simulink model "SEMS_2025_MATLAB file"  (R2024b)
settings: Solver=VariableStepAuto  StartTime=0.0  StopTime=24  RelTol=1e-3
undefined symbols (not defined in the file): Ion, Lithium
libraries: spsSeriesRLCBranchLib x4, spsBatteryLib x1, spsCurrentMeasurementLib x1, spsDiodeLib x1, spsIGBTDiodeLib x1, spsPVArrayLib x1, spsPWMGeneratorDCDCLib x1, spsVoltageMeasurementLib x1, spspowerguiLib x1
settings Model: Creator=sumanth  LastModifiedBy=sumanth

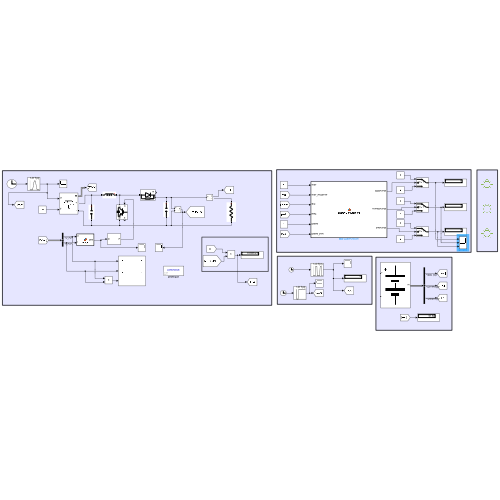
[thumbnail: Simulink's stored preview of the top-level diagram]
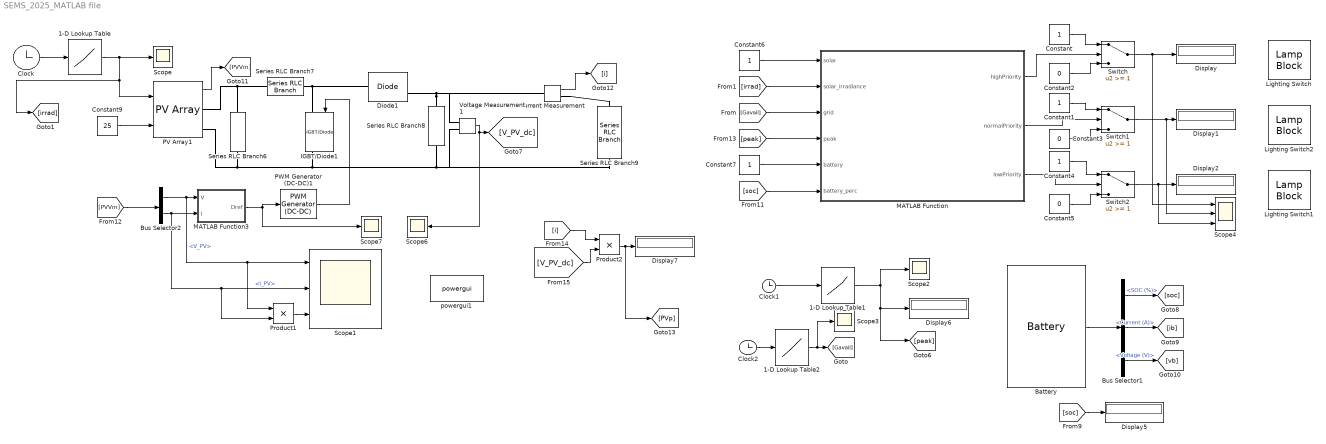
== system SEMS_2025_MATLAB file ==
  1-D Lookup Table : Lookup_n-D  NumberOfTableDimensions=1  BreakpointsForDimension1=[0 1 2 3 4 5 6 7 8 9 10 11 12 13 14 15 16 17 18 19 20 21 22 23]  Table=[0 0 0 0 0 0 0 79 315 533 710 819 855 817 707 532 311 75 0 0 0 0 0 0]  InternalRulePriority=Speed  RndMeth=Simplest
  1-D Lookup Table1 : Lookup_n-D  NumberOfTableDimensions=1  BreakpointsForDimension1=[0 1 2 3 4 5 6 7 8 9 10 11 12 13 14 15 16 17 18 19 20 21 22 23]  Table=[0 0 0 0 0 0 1 1 1 1 0 0 0 0 0 0 0 1 1 1 1 0 0 0]  InternalRulePriority=Speed  RndMeth=Simplest
  1-D Lookup Table2 : Lookup_n-D  NumberOfTableDimensions=1  BreakpointsForDimension1=[0 1 2 3 4 5 6 7 8 9 10 11 12 13 14 15 16 17 18 19 20 21 22 23]  Table=[1 1 0 0 0 0 1 1 1 1 1 1 1 1 1 1 1 1 1 1 1 1 1 1]  InternalRulePriority=Speed  RndMeth=Simplest
  Battery : spsBatteryLib/Battery  BatType=Lithium-Ion  NomV=24  NomQ=50  SOC=50  Batt_Tr=1  PresetModel=on  MaxQ=50  MinV=18  FullV=27.9357  Dis_rate=21.7391  R=0.0048  Normal_OP=45.2174  expZone="[25.9293      2.45652]"
  Bus Selector1 : BusSelector  OutputSignals=SOC (%),Current (A),Voltage (V)
  Bus Selector2 : BusSelector  OutputSignals=V_PV,I_PV
  Clock : Clock
  Clock1 : Clock
  Clock2 : Clock
  Constant{,1,4,6..7} (5 alike) : Constant
  Constant2 : Constant  Value=0
  Constant3 : Constant  Value=0
  Constant5 : Constant  Value=0
  Constant9 : Constant  Value=25
  Current Measurement : spsCurrentMeasurementLib/Current Measurement  PhasorSimulation=off  OutputType=Complex  PSBequivalent=0
  Diode1 : spsDiodeLib/Diode  Ron=0.001  Lon=0  Vf=0.8  IC=0  UseSnubber=0  Rs=500  Cs=250e-9  Measurements=on
  Display{,1..2,5..7} (6 alike) : Display
  IGBT/Diode1 : spsIGBTDiodeLib/IGBT//Diode  Ron=1e-3  Rs=1e5  Cs=inf  Measurements=on
  Lighting Switch : LampBlock  LabelPosition=Hide  Icon=LightingSwitch
  Lighting Switch1 : LampBlock  LabelPosition=Hide  Icon=LightingSwitch
  Lighting Switch2 : LampBlock  LabelPosition=Hide  Icon=LightingSwitch
  MATLAB Function : MATLAB Function  TreatAsAtomicUnit=on
  MATLAB Function3 : MATLAB Function  TreatAsAtomicUnit=on
  PV Array1 : spsPVArrayLib/PV Array  Npar=1300  Nser=11  PlotType=array @ 25 deg.C & specified irradiances  S_vec="[ 1000  500  100 ]"  Temp_C_vec="[ 45 25  ]"  ModuleName=User-defined  PlotWhenSelected=off  Pm=213.15  Ncell=60  Voc=36.3  Isc=7.84  Vm=29  Im=7.35  beta_Voc_pc=-0.36099  alpha_Isc_pc=0.102  beta_Voc=-0.13104  alpha_Isc=0.0079968  IL=7.8654  I0=2.9273e-10  nI=0.98119  Rsh=313.0553  Rs=0.39381  RobustModel=off  RobustCellTemperature=313.3991  BAL=on  Tc=1e-6  Tfilter=5e-5
  PWM Generator (DC-DC)1 : spsPWMGeneratorDCDCLib/PWM Generator (DC-DC)  Fsw=10000  Ts=0
  Product1 : Product
  Product2 : Product
  Scope{,2..3,6..7} (5 alike) : Scope
  Scope1 : Scope  NumInputPorts=3
  Scope4 : Scope  NumInputPorts=3
  Series RLC Branch6 : spsSeriesRLCBranchLib/Series RLC Branch  LConnTagsString=__new0  RConnTagsString=__new0  BranchType=C  Resistance=1  Inductance=1e-3  SetiL0=off  InitialCurrent=0  Capacitance=0.0397  Setx0=off  InitialVoltage=0  Measurements=None
  Series RLC Branch7 : spsSeriesRLCBranchLib/Series RLC Branch  LConnTagsString=__new0  RConnTagsString=__new0  BranchType=L  Resistance=1  Inductance=1.5636e-4  SetiL0=off  InitialCurrent=0  Capacitance=1e-6  Setx0=off  InitialVoltage=0  Measurements=None
  Series RLC Branch8 : spsSeriesRLCBranchLib/Series RLC Branch  LConnTagsString=__new0  RConnTagsString=__new0  BranchType=C  Resistance=1  Inductance=1e-3  SetiL0=off  InitialCurrent=0  Capacitance=0.0397  Setx0=off  InitialVoltage=0  Measurements=None
  Series RLC Branch9 : spsSeriesRLCBranchLib/Series RLC Branch  LConnTagsString=__new0  RConnTagsString=__new0  BranchType=R  Resistance=1  Inductance=1e-3  SetiL0=off  InitialCurrent=0  Capacitance=1e-6  Setx0=off  InitialVoltage=0  Measurements=None
  Switch : Switch  Threshold=1  SaturateOnIntegerOverflow=off  InputSameDT=off
  Switch1 : Switch  Threshold=1  SaturateOnIntegerOverflow=off  InputSameDT=off
  Switch2 : Switch  Threshold=1  SaturateOnIntegerOverflow=off  InputSameDT=off
  Voltage Measurement1 : spsVoltageMeasurementLib/Voltage Measurement  PhasorSimulation=off  OutputType=Complex  PSBequivalent=0
  powergui1 : spspowerguiLib/powergui  Priority=1  SimulationMode=Continuous  SampleTime=50e-6  frequency=60  Iterations=50  frequencyindice=0  Pbase=100e6  ErrMax=1e-4  UnitsV=kV  UnitsW=MW  buscounter=0  FunctionMessages=off  echomessages=off  EnableUseOfTLC=off  CurrentSourceSwitches=off  DisableSnubberDevices=off  DisableRonSwitches=off  DisableVfSwitches=off  DisplayEquations=off  AutomaticDiscreteSolvers=off  SolverType=Tustin/Backward Euler (TBE)  Interpol=off  ExternalGateDelay=off  methode=off  Ts=100  x0status=blocks  SPID=on  SwTol=0  HookPort=off  NonlinearTolerance=1e-4  nMaxIteration=100  ContinueOnMaxIteration=off  RestoreLinks=warning  ResistiveCurrentMeasurement=off  Frange=[0:2:500]  Ylog=off  Xlog=on  ShowGrid=off  save=off  variable=ZData  structure=0  ZoomFFT=off  StartTime=0.0  cycles=1  DisplayStyle=1  fundamental=60  FreqAxis=off  MaxFrequency=1000  frequencyindicesteady=1  RmsSteady=1  display=off
  wires:
  [soc] -> Display5/1
  MATLAB Function/2(normalPriority) -> Switch1/2
  PV Array1/1 -> [PVVm]
  Switch/1 -> Scope4/1, Display/1
  Battery/1 -> Bus Selector1/1
  Switch2/1 -> Scope4/3, Display2/1
  [soc] -> MATLAB Function/6(battery_perc)
  Current Measurement/1 -> [i]
  Product1/1 -> Scope1/3
  Constant/1 -> Switch/1
  Constant2/1 -> Switch/3
  Bus Selector1/1 -> [soc]  "<SOC (%)>"
  MATLAB Function/3(lowPriority) -> Switch2/2
  [peak] -> MATLAB Function/4(peak)
  Constant7/1 -> MATLAB Function/5(battery)
  Bus Selector2/1 -> Product1/1, Scope1/1, MATLAB Function3/1(V)  "<V_PV>"
  Constant6/1 -> MATLAB Function/1(solar)
  Constant3/1 -> Switch1/3
  [PVVm] -> Bus Selector2/1
  [i] -> Product2/1
  Constant5/1 -> Switch2/3
  Bus Selector1/3 -> [vb]  "<Voltage (V)>"
  MATLAB Function/1(highPriority) -> Switch/2
  Switch1/1 -> Scope4/2, Display1/1
  Constant1/1 -> Switch1/1
  Constant4/1 -> Switch2/1
  Bus Selector2/2 -> Product1/2, Scope1/2, MATLAB Function3/2(I)  "<I_PV>"
  MATLAB Function3/1(Dref) -> PWM Generator (DC-DC)1/1, Scope7/1
  Product2/1 -> [PVp], Display7/1
  PWM Generator (DC-DC)1/1 -> IGBT/Diode1/1
  Voltage Measurement1/1 -> [V_PV_dc], Scope6/1
  Constant9/1 -> PV Array1/2
  Bus Selector1/2 -> [ib]  "<Current (A)>"
  [V_PV_dc] -> Product2/2
  Clock/1 -> 1-D Lookup Table/1
  1-D Lookup Table1/1 -> [peak], Display6/1, Scope2/1
  Clock1/1 -> 1-D Lookup Table1/1
  1-D Lookup Table2/1 -> Scope3/1, [Gavail]
  Clock2/1 -> 1-D Lookup Table2/1
  [Gavail] -> MATLAB Function/3(grid)
  1-D Lookup Table/1 -> [irrad], PV Array1/1, Scope/1
  [irrad] -> MATLAB Function/2(solar_irradiance)
  connections:
  Series RLC Branch8/LConn1 -- Diode1/RConn1 -- Current Measurement/LConn1 -- Voltage Measurement1/LConn1
  Series RLC Branch6/LConn1 -- Series RLC Branch7/RConn1 -- PV Array1/RConn1
  Series RLC Branch8/RConn1 -- Series RLC Branch9/RConn1 -- Voltage Measurement1/LConn2 -- IGBT/Diode1/RConn1 -- PV Array1/RConn2 -- Series RLC Branch6/RConn1
  Diode1/LConn1 -- IGBT/Diode1/LConn1 -- Series RLC Branch7/LConn1
  Current Measurement/RConn1 -- Series RLC Branch9/LConn1

== matlab function SEMS_2025_MATLAB file/MATLAB Function ==
  data: solar input; solar_irradiance input; highPriority output; grid input; peak input; normalPriority output; battery input; lowPriority output; battery_perc input
function [highPriority, normalPriority, lowPriority] = energyManagement(solar,solar_irradiance,grid,peak, battery,battery_perc)
    highPriority = 0;
    normalPriority = 0;
    lowPriority = 0;
    if solar == 1 && solar_irradiance >=500
        if solar_irradiance >=700
            highPriority = 1;
            normalPriority = 1;
            lowPriority = 1;
        else
            highPriority = 1;
            normalPriority = 1;
            lowPriority = 0;
        end
    elseif grid > 0
        if peak==1
            highPriority = 1;
            normalPriority = 1;
            lowPriority = 0;
        else
            highPriority = 1;
            normalPriority = 1;
            lowPriority = 1;
        end
    elseif battery == 1 
        if battery_perc<45
            highPriority = 1;
            normalPriority = 0;
            lowPriority = 0;
        else
            highPriority = 1;
            normalPriority = 1;
            lowPriority = 0;
        end
    elseif grid>0 && battery==1
        if peak<1
            highPriority = 1;
            normalPriority = 1;
            lowPriority = 1;
        else
            highPriority = 1;
            normalPriority = 1;
            lowPriority = 0;
        end
    else
        highPriority = 0;
        normalPriority = 0;
        lowPriority = 0;
    end
end

== matlab function SEMS_2025_MATLAB file/MATLAB Function3 ==
  settings: updateMethod=DISCRETE
  data: V input; Dref output; I input
function Dref=mppt(V,I)
Dinit=0.42;
Dmax=0.9;
Dmin=0.1;
delDref=0.00008;

persistent Vold Pold Drefold

if(isempty(Vold))
    Vold=0;
    Pold=0;
    Drefold=Dinit;
end

P=V*I;
delv=V-Vold;
delp=P-Pold;

if delp>0
    if delv>0
        Dref=Drefold-delDref;
    else
        Dref=Drefold+delDref;
    end
elseif delp<0
    if delv>0
        Dref=Drefold+delDref;
    else
        Dref=Drefold-delDref;
    end
else
    Dref=Drefold;
end

if Dref>Dmax || Dref<Dmin
    Dref=Drefold;
end

Drefold=Dref;
Pold=P;
Vold=V;
